simulink model "VTOL_v2_r2018b"  (R2018b)
settings: Solver=FixedStepAuto  StartTime=0.0  StopTime=inf  FixedStep=Ts  RelTol=1e-3  EnableMultiTasking=on
values from neighbouring files (symbols this model uses):
  deltaprops = 0*0.11/2    (= 0)    [VTOL_params.m]
  Ts = 1/10    (= 0.1)    [VTOL_params.m]
undefined symbols (not defined in the file or in its folder): dev, Main, pwm_output0
libraries: aerolibutil x7, px4uORBlib x4, pwm_sig_converters x4, px4Sensorslib x3, simulink x3, px4lib x1, sharedtransform x1
(part 1 of 2)
settings Model: SimulationMode=external  ExtModeTrigDuration=10  Creator=Robert  LastModifiedBy=Robert
settings SolverCC: PositivePriorityOrder=on
settings DataIOCC: SaveOutput=off  SignalLogging=off  DSMLogging=off  SaveTime=off
settings OptimizationCC: DefaultUnderspecifiedDataType=single  EnhancedBackFolding=on  PassReuseOutputArgsAs=Individual arguments  MaxStackSize=64  OptimizeBlockOrder=speed  DifferentSizesBufferReuse=on  OptimizationCustomize=off
settings DebuggingCC: ParameterTunabilityLossMsg=error
settings HardwareCC: ProdBitPerPointer=32  ProdBitPerSizeT=32  ProdBitPerPtrDiffT=32  ProdLargestAtomicInteger=Long  ProdLargestAtomicFloat=Double  ProdWordSize=32  ProdLongLongMode=on  ProdHWDeviceType=ARM Compatible->ARM Cortex
settings SFSimCC: MATLABDynamicMemAlloc=off
settings RTWCC: SystemTargetFile=ert.tlc  HardwareBoard=PX4 Pixhawk 1  TLCOptions="-aInlineSetEventsForThisBaseRateFcn=TLC_FALSE -aSuppressMultiTaskScheduler=TLC_FALSE  -aRateBasedStepFcn=0"  TemplateMakefile=ert_default_tmf  GenerateReport=on  Toolchain=GNU Tools for PX4 Autopilots  BuildConfiguration=Faster Runs  IncludeHyperlinkInReport=on  LaunchReport=on  TargetLang=C++  GenerateTraceInfo=on  GenerateTraceReport=on  GenerateTraceReportSl=on  GenerateTraceReportSf=on  GenerateTraceReportEml=on
settings CodeAppCC: ForceParamTrailComments=on  IgnoreCustomStorageClasses=off  OperatorAnnotations=on  SimulinkDataObjDesc=on  SFDataObjDesc=on  InsertBlockDesc=on

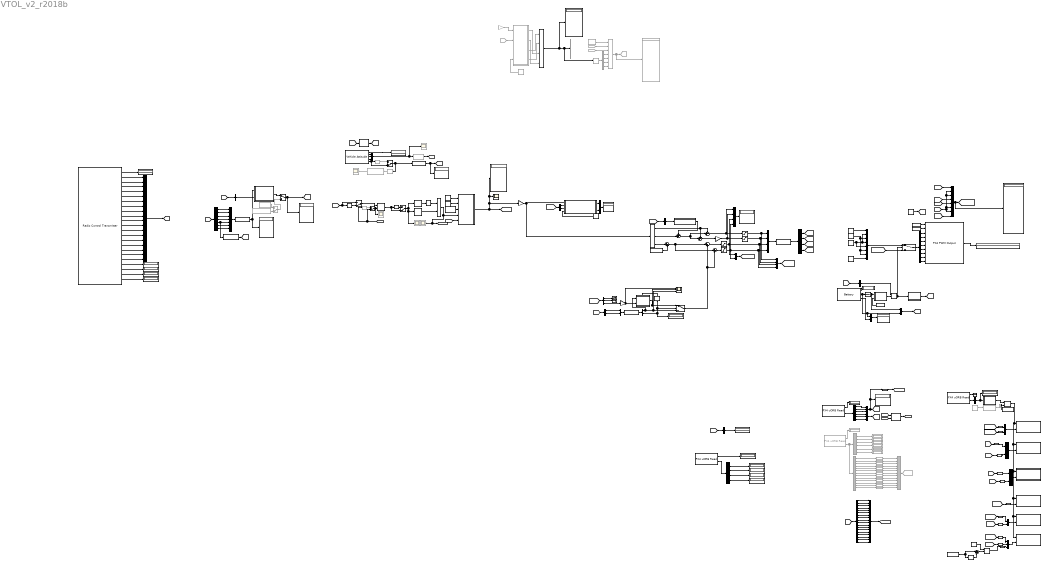
== system VTOL_v2_r2018b ==
  note: The PID parameters for roll/pitch on the single engine one
      | that works are approx
      | [0.6,0,0.015;
      |  0.6,0,0.015]
      |
      | That is, P/D = 40
  note: Some constant pitch torque offset
      | may be necessary due to c.g. z-offset. (No integrators in controller)
  note: Control Area
  note: Before Torque-Translator is used, lets make sure we can hover with this simple linear mixer.
      | Working around the hover point does not need the full range and thus complete non-linear controller.
      | Basic tuning is easier this way - less parameters to adjust.
  note: Part 2 of 2 of the heart of this project.
      | Once the Pixhawk is stable and hover works acceptable this part will be inserted, normalized to not
      | alter the behaviour too much at hover mode, and extend the responses to work well in flying and
      | transition mode as well.
  note: Old translator, only kept for code reference, will never be used.
  note: Crude, ad-hoc, altitude holder for the hover mode.
      | Far from perfect but does the job and frees up one hand to trim/adjust setting etc while hovering.
      | When not holding alt => Pass through
      | throttle stick to joint thrust.
  note: Generate reference quaternion from Transmitter inputs. Very crude reference now, but enough to test stability and do some small steps.
      | Verified in external mode with manual switches.
      |
      | The "mode" (bottom) selects absolute/rate mode
      | on input..
  note: Quaternion extraction from EKF.
      | Handedness verified with manual switches in external mode.
  note: Debug safety switch status
  note: lowpass filter batt voltage for
      | more accurate shutoffs
  note: 3V/cell in LiPo is absolutely the lowest allowed
  note: Make sure model runs at specified frequency
  note: Above (commented out) was a work-around before I got the
      | fixed code for the log block to log at every time step.
  note: Props may not be symmetrical, this offsets the thrust to compensate in that case.
  note: Emergency shutdown switch forces things into
      | off or neutral
  note: Inputs from RC
  note: Outputs, to Servos
  note: Emil Fresk paper on quaternion control, this is part 1 of 2 of the focus on this project. Originally a non-linear attitude controller for
      | multi-rotors, I am trying to use it as a controller for a VTOL fixed wing, non vectored along with a sensitivity normalizer
      | to allow a single controller for hover, transitioning and flying modes.
  note: If either manual emergency stop is pressed or voltage too low cut power.
  note: Logging to SD
  AND : Logic  IconShape=distinctive  AllPortsSameDT=off  OutDataTypeStr=boolean
  Battery : px4Sensorslib/Battery  voltage=on  current=off  remaining=on  warning=off  timestamp=off  sampleTime=Ts  BlockingMode=off  BlockTimeout=1e-3
      settings: SourceProductName=Embedded Coder Support Package for PX4 Autopilots
  Bus Creator : BusCreator  Inputs=18
  Bus Selector : BusSelector  OutputSignals=ch9_SC
  Bus Selector1 : BusSelector  OutputSignals=safety_switch_available,safety_off,override_available,override_enabled
  Bus Selector10 : BusSelector  Commented=on  OutputSignals=fix_type,satellites_used,lat,lon,alt,hdop,vdop,noise_per_ms,jamming_indicator,vel_m_s,vel_n_m_s,vel_e_m_s,vel_d_m_s
  Bus Selector11 : BusSelector  OutputSignals=ch10_SD
  Bus Selector12 : BusSelector  OutputSignals=ch5_S1
  Bus Selector13 : BusSelector  OutputSignals=safety_off
  Bus Selector2 : BusSelector  OutputSignals=ch5_S1
  Bus Selector3 : BusSelector  OutputSignals=ch1_thrust,ch2_Ail,ch3_Ele,ch4_Rud,ch8_SB,ch6_S2,ch7_SA
  Bus Selector6 : BusSelector  OutputSignals=x,y,z,vx,vy,vz
  Bus Selector7 : BusSelector  OutputSignals=ch1_thrust,ch2_Ail,ch3_Ele,ch4_Rud,ch5_S1,ch6_S2,ch7_SA,ch8_SB,ch9_SC,ch10_SD,ch11_SE,ch12_SF,ch13_SG,ch14_SH,ch15_LS,ch16_RS,ch17_MAX,ch18_MIN
  Bus Selector8 : BusSelector  Commented=on  OutputSignals=lat,lon,alt,satellites_used,hdop,vdop
  Bus Selector9 : BusSelector  OutputSignals=ch1_thrust,ch12_SF
  Cast To Boolean : DataTypeConversion  Commented=on  OutDataTypeStr=boolean
  Compare To Zero : simulink/Logic and Bit Operations/Compare To Zero  relop=>  OutDataTypeStr=boolean
  Constant : Constant  Value=logical(1)
  Constant1 : Constant  Value=logical(0)
  Constant10 : Constant  Value=1500  OutDataTypeStr=uint16
  Constant11 : Constant  Value=1500  OutDataTypeStr=uint16
  Constant12 : Constant  Value=1500  OutDataTypeStr=uint16  SampleTime=Ts
  Constant13 : Constant  Commented=on  Value=[cos(pi/4),0,sin(pi/4),0]  SampleTime=Ts
  Constant14 : Constant  Value=boolean(true)  SampleTime=Ts
  Constant16 : Constant  SampleTime=Ts
  Constant17 : Constant  Value=[2,4,1]'  VectorParams1D=off  SampleTime=Ts
  Constant2 : Constant  Commented=on  Value=[0,0,0]  OutDataTypeStr=single  SampleTime=Ts
  Constant3 : Constant  Commented=on  Value=0  SampleTime=Ts
  Constant4 : Constant  Value=0.015  SampleTime=Ts
  Constant5 : Constant  Value=0.6  SampleTime=Ts
  Constant6 : Constant  Value=[0,0,0]  SampleTime=Ts
  Constant7 : Constant  Value=1500  OutDataTypeStr=uint16
  Constant8 : Constant  Commented=on  Value=[1,0,0,0]  SampleTime=Ts
  Constant9 : Constant  Value=900  OutDataTypeStr=uint16
  CutoffVoltage : Constant  Value=3.0*3  OutDataTypeStr=single  SampleTime=Ts
  Data Type Conversion{4..16} (13 alike) : DataTypeConversion  Commented=on  OutDataTypeStr=single
  Data Type Conversion{2..3,17,20..26,28} (11 alike) : DataTypeConversion  OutDataTypeStr=single
  Data Type Conversion18 : DataTypeConversion  OutDataTypeStr=uint16
  Data Type Conversion19 : DataTypeConversion  OutDataTypeStr=uint16
  Data Type Conversion27 : DataTypeConversion  Commented=on  OutDataTypeStr=double
  Demux : Demux  Outputs=8
  Demux1 : Demux  Commented=on
  Demux4 : Demux  Commented=on
  Demux5 : Demux  Outputs=3
  Demux6 : Demux  Outputs=2
  Demux7 : Demux  Outputs=3
  Demux8 : Demux  Outputs=2
  Demux9 : Demux
  Digital Clock1 : DigitalClock  SampleTime=Ts
  Discrete Transfer Fcn : DiscreteTransferFcn  Numerator=[1-0.99]  Denominator=[1 -0.99]  SampleTime=Ts
  Display{,1..2,4..15,22,26..27,33..41} (27 alike) : Display
      Display9 settings: Format=binary (Stored Integer)
  Display{20..21,23,28..32} (8 alike) : Display  Commented=on
  Divide1 : Product  Inputs=*/
  From15 : From  Commented=on  GotoTag=w_bf
  From16 : From  Commented=on  GotoTag=q_bf
  From21 : From  Commented=on  GotoTag=states
  Gain1 : Gain  Commented=on  Gain=18
  Gain2 : Gain
  Gain3 : Gain  Gain=-1
  Gain4 : Gain  Gain=-1
  Goto11 : Goto  Commented=on  GotoTag=states
  Goto25 : Goto  Commented=on  GotoTag=GPSinfo
  MATLAB Function11 : MATLAB Function  TreatAsAtomicUnit=on
  MATLAB Function12 : MATLAB Function  TreatAsAtomicUnit=on
  MATLAB Function14 : MATLAB Function  TreatAsAtomicUnit=on
  MATLAB Function15 : MATLAB Function  TreatAsAtomicUnit=on
  MATLAB Function16 : MATLAB Function  TreatAsAtomicUnit=on
  MATLAB Function17 : MATLAB Function  TreatAsAtomicUnit=on
  MATLAB Function18 : MATLAB Function  TreatAsAtomicUnit=on
  Manual Switch{,1..3} (4 alike) : ManualSwitch  CurrentSetting=0
  Manual Switch4 : ManualSwitch
  Manual Switch5 : ManualSwitch  Commented=on  CurrentSetting=0
  Max : MinMax  Function=max  Inputs=2  OutDataTypeStr=uint16
  Memory : Memory  Commented=on  InheritSampleTime=on
  Memory2 : Memory  InheritSampleTime=on
  Multiply : Product
  Mux : Mux  Inputs=7
  Mux10 : Mux  Commented=on  Inputs=7
  Mux{11..12,17..20,22..23,26} (9 alike) : Mux  Inputs=2
  Mux13 : Mux  Commented=on  Inputs=13
  Mux14 : Mux  Inputs=8
  Mux{2,16,24,27} (4 alike) : Mux
  Mux21 : Mux  Inputs=8
  Mux{5..7,25} (4 alike) : Mux  Inputs=3
  Mux8 : Mux  Inputs=18
  PX4 PWM Output : px4lib/PX4 PWM Output  pwmDevice=Main (/dev/pwm_output0)  pwmChannel1_=on  pwmChannel2_=on  pwmChannel3_=on  pwmChannel4_=on  pwmChannel5_=on  pwmChannel6_=on  pwmChannel7_=on  pwmChannel8_=on  forceTerminateFailsafe=off  outputErrorStatus=on
      settings: SourceProductName=Embedded Coder Support Package for PX4 Autopilots
  PX4 SD Card Logger1 : Subsystem  mask(PX4 SD Card Logger){logfile=/fs/microsd/log, logfilename=qlogs, cacheflag=off, numRecs=250*60*60}
      mask prompts: logfile "Log Folder"; logfilename "Log File Name"; cacheflag "Cache in Memory"; numRecs "Maximum Record Count"
      mask help:
      | Log data to a specified file on the SD card
      |
      | The block accepts two inputs, enable and data. The incoming data is logged into the SD card when the enable signal is high and the number of data points logged is less than the Maximum Record Count specified.
      |
      | The specified folder should be present in the SD card for logging.
      |
      | If Cache in Memory is unchecked, the data is written to the SD card at every timestep.  If Cache in Memory is checked, data is cached in the memory and is written to SD card only when enable goes low or when the number of data points logged reaches the Maximum Record Count specified.
      mask init:
      | logname=uint8([logfile,'/',logfilename]);
      mask Help: eval('codertarget.internal.helpView(''px4'',''px4sdcardexample'')');
      mask Display:
      | fprintf([get_param(gcb,'logfile'),'/',get_param(gcb,'logfilename')])
      | port_label('input',1,'en')
      | port_label('input',2,'data')
  PX4 SD Card Logger2 : Subsystem  mask(PX4 SD Card Logger){logfile=/fs/microsd/log, logfilename=rc_and_servosignals, cacheflag=off, numRecs=250*60*60}
      mask prompts: logfile "Log Folder"; logfilename "Log File Name"; cacheflag "Cache in Memory"; numRecs "Maximum Record Count"
      mask help:
      | Log data to a specified file on the SD card
      |
      | The block accepts two inputs, enable and data. The incoming data is logged into the SD card when the enable signal is high and the number of data points logged is less than the Maximum Record Count specified.
      |
      | The specified folder should be present in the SD card for logging.
      |
      | If Cache in Memory is unchecked, the data is written to the SD card at every timestep.  If Cache in Memory is checked, data is cached in the memory and is written to SD card only when enable goes low or when the number of data points logged reaches the Maximum Record Count specified.
      mask init:
      | logname=uint8([logfile,'/',logfilename]);
      mask Help: eval('codertarget.internal.helpView(''px4'',''px4sdcardexample'')');
      mask Display:
      | fprintf([get_param(gcb,'logfile'),'/',get_param(gcb,'logfilename')])
      | port_label('input',1,'en')
      | port_label('input',2,'data')
  PX4 SD Card Logger3 : Subsystem  mask(PX4 SD Card Logger){logfile=/fs/microsd/log, logfilename=norm_sigs, cacheflag=off, numRecs=250*60*60}
      mask prompts: logfile "Log Folder"; logfilename "Log File Name"; cacheflag "Cache in Memory"; numRecs "Maximum Record Count"
      mask help:
      | Log data to a specified file on the SD card
      |
      | The block accepts two inputs, enable and data. The incoming data is logged into the SD card when the enable signal is high and the number of data points logged is less than the Maximum Record Count specified.
      |
      | The specified folder should be present in the SD card for logging.
      |
      | If Cache in Memory is unchecked, the data is written to the SD card at every timestep.  If Cache in Memory is checked, data is cached in the memory and is written to SD card only when enable goes low or when the number of data points logged reaches the Maximum Record Count specified.
      mask init:
      | logname=uint8([logfile,'/',logfilename]);
      mask Help: eval('codertarget.internal.helpView(''px4'',''px4sdcardexample'')');
      mask Display:
      | fprintf([get_param(gcb,'logfile'),'/',get_param(gcb,'logfilename')])
      | port_label('input',1,'en')
      | port_label('input',2,'data')
  PX4 SD Card Logger4 : Subsystem  mask(PX4 SD Card Logger){logfile=/fs/microsd/log, logfilename=MainLog, cacheflag=off, numRecs=250*60*60}
      mask prompts: logfile "Log Folder"; logfilename "Log File Name"; cacheflag "Cache in Memory"; numRecs "Maximum Record Count"
      mask help:
      | Log data to a specified file on the SD card
      |
      | The block accepts two inputs, enable and data. The incoming data is logged into the SD card when the enable signal is high and the number of data points logged is less than the Maximum Record Count specified.
      |
      | The specified folder should be present in the SD card for logging.
      |
      | If Cache in Memory is unchecked, the data is written to the SD card at every timestep.  If Cache in Memory is checked, data is cached in the memory and is written to SD card only when enable goes low or when the number of data points logged reaches the Maximum Record Count specified.
      mask init:
      | logname=uint8([logfile,'/',logfilename]);
      mask Help: eval('codertarget.internal.helpView(''px4'',''px4sdcardexample'')');
      mask Display:
      | fprintf([get_param(gcb,'logfile'),'/',get_param(gcb,'logfilename')])
      | port_label('input',1,'en')
      | port_label('input',2,'data')
  PX4 SD Card Logger5 : Subsystem  mask(PX4 SD Card Logger){logfile=/fs/microsd/log, logfilename=torques, cacheflag=off, numRecs=250*60*60}
      mask prompts: logfile "Log Folder"; logfilename "Log File Name"; cacheflag "Cache in Memory"; numRecs "Maximum Record Count"
      mask help:
      | Log data to a specified file on the SD card
      |
      | The block accepts two inputs, enable and data. The incoming data is logged into the SD card when the enable signal is high and the number of data points logged is less than the Maximum Record Count specified.
      |
      | The specified folder should be present in the SD card for logging.
      |
      | If Cache in Memory is unchecked, the data is written to the SD card at every timestep.  If Cache in Memory is checked, data is cached in the memory and is written to SD card only when enable goes low or when the number of data points logged reaches the Maximum Record Count specified.
      mask init:
      | logname=uint8([logfile,'/',logfilename]);
      mask Help: eval('codertarget.internal.helpView(''px4'',''px4sdcardexample'')');
      mask Display:
      | fprintf([get_param(gcb,'logfile'),'/',get_param(gcb,'logfilename')])
      | port_label('input',1,'en')
      | port_label('input',2,'data')
  PX4 SD Card Logger6 : Subsystem  mask(PX4 SD Card Logger){logfile=/fs/microsd/log, logfilename=volt_stop, cacheflag=off, numRecs=250*60*60}
      mask prompts: logfile "Log Folder"; logfilename "Log File Name"; cacheflag "Cache in Memory"; numRecs "Maximum Record Count"
      mask help:
      | Log data to a specified file on the SD card
      |
      | The block accepts two inputs, enable and data. The incoming data is logged into the SD card when the enable signal is high and the number of data points logged is less than the Maximum Record Count specified.
      |
      | The specified folder should be present in the SD card for logging.
      |
      | If Cache in Memory is unchecked, the data is written to the SD card at every timestep.  If Cache in Memory is checked, data is cached in the memory and is written to SD card only when enable goes low or when the number of data points logged reaches the Maximum Record Count specified.
      mask init:
      | logname=uint8([logfile,'/',logfilename]);
      mask Help: eval('codertarget.internal.helpView(''px4'',''px4sdcardexample'')');
      mask Display:
      | fprintf([get_param(gcb,'logfile'),'/',get_param(gcb,'logfilename')])
      | port_label('input',1,'en')
      | port_label('input',2,'data')
  PX4 uORB Read : px4uORBlib/PX4 uORB Read  uORBTopic=vehicle_local_position  sampleTime=Ts  BlockingMode=off  BlockTimeout=1e-3
      settings: SourceProductName=Embedded Coder Support Package for PX4 Autopilots
  PX4 uORB Read1 : px4uORBlib/PX4 uORB Read  uORBTopic=safety  sampleTime=Ts  BlockingMode=off  BlockTimeout=1e-3
      settings: SourceProductName=Embedded Coder Support Package for PX4 Autopilots
  PX4 uORB Read2 : px4uORBlib/PX4 uORB Read  Commented=on  uORBTopic=vehicle_gps_position  sampleTime=0.004  BlockingMode=off  BlockTimeout=1e-3
      settings: SourceProductName=Embedded Coder Support Package for PX4 Autopilots
  PX4 uORB Read3 : px4uORBlib/PX4 uORB Read  uORBTopic=safety  sampleTime=Ts  BlockingMode=off  BlockTimeout=1e-3
      settings: SourceProductName=Embedded Coder Support Package for PX4 Autopilots
  PropOffset : Constant  Value=deltaprops  OutDataTypeStr=single  SampleTime=Ts
  Pulse Generator : DiscretePulseGenerator  Commented=on  SampleTime=Ts
  Quaternion Conjugate1 : aerolibutil/Quaternion Conjugate
      settings: SourceProductName=Aerospace Blockset  SourceProductBaseCode=AE
  Quaternion Conjugate10 : aerolibutil/Quaternion Conjugate
      settings: SourceProductName=Aerospace Blockset  SourceProductBaseCode=AE
  Quaternion Conjugate2 : aerolibutil/Quaternion Conjugate  Commented=on
      settings: SourceProductName=Aerospace Blockset  SourceProductBaseCode=AE
  Quaternion Conjugate7 : aerolibutil/Quaternion Conjugate  Commented=on
      settings: SourceProductName=Aerospace Blockset  SourceProductBaseCode=AE
  Quaternion Conjugate8 : aerolibutil/Quaternion Conjugate
      settings: SourceProductName=Aerospace Blockset  SourceProductBaseCode=AE
  Quaternion Multiplication : aerolibutil/Quaternion Multiplication
  Quaternion Rotation4 : aerolibutil/Quaternion Rotation
  Quaternions to Rotation Angles1 : sharedtransform/Quaternions to Rotation Angles  Commented=on  rotationOrder=ZYX  aMode=aMode
      settings: SourceProductBaseCode=AE
  Radio Control Transmitter : px4Sensorslib/Radio Control Transmitter  channel1=on  channel2=on  channel3=on  channel4=on  channel5=on  channel6=on  channel7=on  channel8=on  channel9=on  channel10=on  channel11=on  channel12=on  channel13=on  channel14=on  channel15=on  channel16=on  channel17=on  channel18=on  channel_count=on  rssi=on  rc_input_source=on  timestamp_last_signal=on  time_stamp=off  sampleTime=Ts  BlockingMode=off  BlockTimeout=5
      settings: SourceProductName=Embedded Coder Support Package for PX4 Autopilots
  Saturation{,1..3} (4 alike) : Saturate  UpperLimit=1  LowerLimit=-1
  Scope : Scope  NumInputPorts=3
  Scope{4..6,25,35} (5 alike) : Scope  Commented=on
  Scope7 : Scope
  Selector2 : Selector  IndexMode=Zero-based  InputPortWidth=4  IndexOptions=Index vector (dialog)  Indices=[0 ]  OutputSizes=1
  Selector3 : Selector  IndexMode=Zero-based  InputPortWidth=4  IndexOptions=Index vector (dialog)  Indices=[1:3]  OutputSizes=1
  Sign : Signum
  Signal Specification1 : SignalSpecification  OutDataTypeStr=single
  Subsystem : Subsystem
  Sum2 : Sum  Inputs=-+|
  Sum3 : Sum  Inputs=++|
  Sum4 : Sum  Inputs=|++
  Sum5 : Sum  Inputs=|-+
  Sum6 : Sum  Inputs=++|
  Sum7 : Sum  Inputs=|++
  Sum9 : Sum  Inputs=|+-
  Switch : Switch  Criteria=u2 > Threshold
  Switch1 : Switch  Criteria=u2 > Threshold  Threshold=1300
  Terminator : Terminator
  Terminator1 : Terminator
  Terminator2 : Terminator
  TorqueTranslator : MATLAB Function  Commented=on  TreatAsAtomicUnit=on
  Transfer Fcn First Order1 : simulink/Discrete/Transfer Fcn First Order  Commented=through  PoleZ=0.9  ICPrevOutput=0.0  DoSatur=off
      settings: SourceProductName=Simulink
  Vehicle Attitude1 : px4Sensorslib/Vehicle Attitude  rollRate=on  pitchRate=on  yawRate=on  quaternion=on  uorbTimeStamp=off  BlockingMode=off  BlockTimeout=0.001  sampleTime=Ts
      settings: SourceProductName=Embedded Coder Support Package for PX4 Autopilots
  pwm2sig : pwm_sig_converters/pwm2sig  SystemSampleTime=-1
  pwm2sig1 : pwm_sig_converters/pwm2sig  SystemSampleTime=-1
  pwm2sig2 : pwm_sig_converters/pwm2sig  SystemSampleTime=-1
  sig2pwm : pwm_sig_converters/sig2pwm  SystemSampleTime=-1
  wires:
  Demux1/4 -> Mux10/7
  Quaternion Conjugate7/1 -> Manual Switch/1
  Demux6/2 -> Display37/1, Switch/2, Compare To Zero/1
  Bus Selector7/10 -> Mux8/10  "<ch10_SD>"
  Sum3/1 -> Gain3/1
  Demux7/2 -> Terminator1/1
  Multiply/1 -> [axis_err], Scope4/1, MATLAB Function11/4(angErr)
  Battery/3 -> Mux22/2
  Demux5/1 -> Sum2/1, Sum3/1  "tao_x"
  [rc_bus] -> Bus Selector11/1
  Switch1/1 -> Demux/1
  Compare To Zero/1 -> Subsystem/Enable
  Battery/2 -> Discrete Transfer Fcn/1, Mux26/2, Mux22/1
  Demux/8 -> PX4 PWM Output/10
  Data Type Conversion8/1 -> Mux13/5
  Constant11/1 -> Mux21/8
  Mux2/1 -> Memory/1, Demux4/1, Display10/1
  Bus Selector/1 -> Display/1  "<ch9_SC>"
  Demux9/2 -> [ElevonR]
  Radio Control Transmitter/16 -> Bus Creator/15  "ch15_LS"
  Demux1/2 -> Mux10/5
  Constant7/1 -> Mux21/1
  Demux/1 -> PX4 PWM Output/3
  Constant9/1 -> Mux21/2, Mux21/4, Mux21/5
  Bus Selector7/2 -> Mux8/2  "<ch2_Ail>"
  Radio Control Transmitter/8 -> Bus Creator/7  "ch7_SA"
  Quaternion Multiplication/1 -> Quaternion Conjugate10/1, Manual Switch3/2  "qerr_wf"
  Demux7/3 -> Gain4/1
  Demux9/4 -> [ThrustR]
  Constant6/1 -> MATLAB Function14/4(v)
  [ServoSignals] -> Switch1/3
  Bus Selector10/2 -> Data Type Conversion5/1  "<satellites_used>"
  Mux20/1 -> Display38/1
  Max/1 -> MATLAB Function18/1(u), Switch1/2
  Sum6/1 -> Sum3/2, Sum2/2
  Bus Selector7/3 -> Mux8/3  "<ch3_Ele>"
  Bus Selector10/6 -> Data Type Conversion9/1  "<hdop>"
  Data Type Conversion6/1 -> Mux13/3
  Subsystem/1("throttle ") -> Switch/1, Scope/2
  Constant10/1 -> Mux21/7, Mux21/6, Mux21/3
  Bus Selector6/5 -> Mux7/2  "<vy>"
  MATLAB Function15/1(stopsig) -> Max/2
  Demux8/1 -> MATLAB Function14/2(u_omegaL)
  Bus Selector3/5 -> pwm2sig2/1, Mux/5  "<ch8_SB>"
  Radio Control Transmitter/19 -> Bus Creator/18  "ch18_MIN"
  Data Type Conversion9/1 -> Mux13/6
  Bus Selector8/4 -> Display21/1  "<satellites_used>"
  TorqueTranslator/3(u_deltaL) -> Mux2/1  "uWL"
  Bus Selector10/10 -> Data Type Conversion13/1  "<vel_m_s>"
  Manual Switch1/1 -> Quaternion Multiplication/1
  Bus Selector6/1 -> Mux5/1  "<x>"
  PX4 PWM Output/1 -> Display9/1
  Gain3/1 -> Mux16/2, Saturation1/1
  Gain2/1 -> MATLAB Function14/1(tao), Demux5/1
  Bus Selector3/6 -> Mux/6  "<ch6_S2>"
  Bus Selector9/1 -> Mux18/1  "<ch1_thrust>"
  Switch/1 -> Sum4/2, Sum5/2
  Mux22/1 -> Display39/1
  Bus Selector11/1 -> Max/1  "<ch10_SD>"
  Radio Control Transmitter/21 -> Display12/1
  Demux6/1 -> Subsystem/1(throttle), Switch/3, Scope/3
  Bus Selector1/3 -> Display6/1  "<override_available>"
  Demux/4 -> PX4 PWM Output/6
  Demux8/2 -> MATLAB Function14/3(u_omegaR)
  Data Type Conversion7/1 -> Mux13/4
  [u_omegas] -> Demux8/1
  Bus Selector10/9 -> Data Type Conversion12/1  "<jamming_indicator>"
  [q_wf] -> Manual Switch/2, Quaternion Conjugate7/1  "qerr_bf"
  Sum7/1 -> Sum5/1, Sum4/1
  Demux/3 -> PX4 PWM Output/5
  Manual Switch4/1 -> [q_ref], Display36/1
  [Position] -> Demux7/1
  Constant2/1 -> Mux10/1
  Bus Selector8/1 -> Display29/1  "<lat>"
  Mux21/1 -> Switch1/1
  Manual Switch3/1 -> Scope35/1, Selector3/1, Selector2/1
  Mux19/1 -> [u_omegas]
  [w_bf] -> MATLAB Function11/5(w)
  Bus Selector7/8 -> Mux8/8  "<ch8_SB>"
  Sign/1 -> Multiply/1  "rotdir"
  Data Type Conversion16/1 -> Mux13/13
  Gain4/1 -> Scope/1, Subsystem/2(alt)
  Vehicle Attitude1/5 -> Manual Switch2/2, Quaternion Conjugate2/1
  Vehicle Attitude1/4 -> Mux6/3
  Radio Control Transmitter/6 -> Bus Creator/5  "ch5_S1"
  [ElevonR] -> Mux14/1
  TorqueTranslator/4(u_deltaR) -> Mux2/2  "udeltaL"
  Vehicle Attitude1/2 -> Mux6/1
  Bus Selector1/1 -> Display4/1  "<safety_switch_available>"
  Quaternion Conjugate1/1 -> [q_bf]
  Constant17/1 -> MATLAB Function11/3(axisgains)
  PX4 uORB Read1/2 -> Bus Selector1/1
  pwm2sig1/1 -> MATLAB Function12/1(sticks), Display35/1
  [rc_bus] -> Bus Selector3/1
  Demux9/3 -> [ThrustL]
  Bus Selector10/11 -> Data Type Conversion14/1  "<vel_n_m_s>"
  Bus Selector6/4 -> Mux7/1  "<vx>"
  Bus Selector3/3 -> Mux/3  "<ch3_Ele>"
  Bus Selector3/1 -> Mux/1  "<ch1_thrust>"
  Bus Selector10/8 -> Data Type Conversion11/1  "<noise_per_ms>"
  Demux9/1 -> [ElevonL]
  Data Type Conversion14/1 -> Mux13/11
  Bus Selector10/12 -> Data Type Conversion15/1  "<vel_e_m_s>"
  Bus Selector7/15 -> Mux8/15  "<ch15_LS>"
  Data Type Conversion12/1 -> Mux13/9
  Data Type Conversion13/1 -> Mux13/10
  Bus Selector7/9 -> Mux8/9  "<ch9_SC>"
  [ThrustL] -> Mux14/5
  Data Type Conversion10/1 -> Mux13/7
  Data Type Conversion5/1 -> Mux13/2
  Demux/6 -> PX4 PWM Output/8
  Selector3/1 -> Multiply/2  "axiserr"
  Demux/7 -> PX4 PWM Output/9
  Mux7/1 -> [v_wf]
  Mux14/1 -> Display8/1, [ServoSignals]
  [Others] -> Mux14/2, Mux14/3, Mux14/6, Mux14/7
  Bus Selector7/12 -> Mux8/12  "<ch12_SF>"
  Radio Control Transmitter/3 -> Bus Creator/2  "ch2_Ail"
  Bus Selector7/14 -> Mux8/14  "<ch14_SH>"
  Bus Selector7/11 -> Mux8/11  "<ch11_SE>"
  Radio Control Transmitter/23 -> Display13/1
  Bus Selector10/1 -> Data Type Conversion4/1  "<fix_type>"
  [rc_bus] -> Bus Selector7/1
  Bus Selector7/6 -> Mux8/6  "<ch6_S2>"
  Bus Selector10/13 -> Data Type Conversion16/1  "<vel_d_m_s>"
  TorqueTranslator/2(u_omegaR) -> Mux2/4
  Bus Selector7/7 -> Mux8/7  "<ch7_SA>"
  [q_wf] -> Quaternion Conjugate1/1
  Manual Switch/1 -> Scope25/1, Quaternion Multiplication/2
  Bus Selector7/18 -> Mux8/18  "<ch18_MIN>"
  Mux16/1 -> Display33/1
  Selector2/1 -> Sign/1  "q0"
  Sum2/1 -> Mux16/1, Saturation/1
  From16/1 -> Mux10/3  "q"
  [q_ref] -> Manual Switch1/1, Quaternion Conjugate8/1
  Vehicle Attitude1/3 -> Mux6/2
  Constant4/1 -> MATLAB Function11/2(D)
  Gain1/1 -> TorqueTranslator/1(u_jointT)
  Data Type Conversion17/1 -> [Position]
  Constant5/1 -> MATLAB Function11/1(P)
  MATLAB Function11/1(taos) -> Display27/1, Scope7/1, Gain2/1, [torques]
  PX4 uORB Read1/1 -> Display1/1
  [v_wf] -> Quaternion Rotation4/2
  Bus Selector7/4 -> Mux8/4  "<ch4_Rud>"
  Bus Selector7/17 -> Mux8/17  "<ch17_MAX>"
  Bus Selector1/2 -> Display5/1  "<safety_off>"
  Sum5/1 -> Saturation3/1
  Bus Selector9/2 -> Mux18/2  "<ch12_SF>"
  Radio Control Transmitter/17 -> Bus Creator/16  "ch16_RS"
  Constant3/1 -> TorqueTranslator/4(pitchoffset)
  From21/1 -> TorqueTranslator/2(states)
  Demux/2 -> PX4 PWM Output/4
  Bus Selector7/16 -> Mux8/16  "<ch16_RS>"
  Memory/1 -> Demux1/1
  Data Type Conversion11/1 -> Mux13/8
  Radio Control Transmitter/11 -> Bus Creator/10  "ch10_SD"
  Sum4/1 -> Saturation2/1
  From15/1 -> Mux10/2  "w"
  TorqueTranslator/1(u_omegaL) -> Mux2/3  "uWL"
  Radio Control Transmitter/20 -> Display11/1
  [ElevonL] -> Mux14/8
  MATLAB Function14/2(u_deltaR) -> Mux20/2
  pwm2sig2/1 -> [mode]
  PX4 uORB Read/1 -> Display34/1
  [ThrustR] -> Mux14/4
  Bus Selector10/4 -> Data Type Conversion7/1  "<lon>"
  Bus Selector3/2 -> Mux/2  "<ch2_Ail>"
  Data Type Conversion4/1 -> Mux13/1
  Quaternion Rotation4/1 -> [v_bf]
  Radio Control Transmitter/14 -> Bus Creator/13  "ch13_SG"
  Signal Specification1/1 -> Display22/1, [q_wf]
  Vehicle Attitude1/1 -> Display26/1
  Bus Selector6/3 -> Mux5/3  "<z>"
  Bus Selector8/2 -> Display30/1  "<lon>"
  PX4 uORB Read/2 -> Bus Selector6/1
  CutoffVoltage/1 -> MATLAB Function15/2(cutoff)
  Radio Control Transmitter/22 -> Display15/1
  Radio Control Transmitter/10 -> Bus Creator/9  "ch9_SC"
  Radio Control Transmitter/15 -> Bus Creator/14  "ch14_SH"
  Radio Control Transmitter/13 -> Bus Creator/12  "ch12_SF"
  Bus Selector7/1 -> Mux8/1  "<ch1_thrust>"
  Radio Control Transmitter/18 -> Bus Creator/17  "ch17_MAX"
  Battery/1 -> Display40/1
  [q_bf] -> Quaternion Rotation4/1
  Mux8/1 -> [RC_inputs]
  Bus Selector10/3 -> Data Type Conversion6/1  "<lat>"
  PX4 uORB Read2/1 -> Display32/1
  Mux18/1 -> pwm2sig/1
  MATLAB Function14/1(u_deltaL) -> Mux20/1
  Radio Control Transmitter/4 -> Bus Creator/3  "ch3_Ele"
  Demux7/1 -> Terminator/1
  Constant1/1 -> PX4 PWM Output/2
  Bus Creator/1 -> [rc_bus]
  Bus Selector1/4 -> Display7/1  "<override_enabled>"
  Bus Selector6/6 -> Mux7/3  "<vz>"
  Radio Control Transmitter/5 -> Bus Creator/4  "ch4_Rud"
  Constant/1 -> PX4 PWM Output/1
  Constant12/1 -> [Others]
  Bus Selector7/5 -> Mux8/5  "<ch5_S1>"
  Demux1/1 -> Mux10/4
  Radio Control Transmitter/1 -> Display14/1
  Radio Control Transmitter/9 -> Bus Creator/8  "ch8_SB"
  [rc_bus] -> Bus Selector/1
  PX4 uORB Read2/2 -> Bus Selector10/1, Bus Selector8/1
  Mux/1 -> pwm2sig1/1
  Radio Control Transmitter/2 -> Bus Creator/1  "ch1_thrust"
  Quaternion Conjugate8/1 -> Manual Switch1/2
  Bus Selector10/5 -> Data Type Conversion8/1  "<alt>"
  Demux1/3 -> Mux10/6
  Bus Selector6/2 -> Mux5/2  "<y>"
  Mux13/1 -> Goto25/1
  Radio Control Transmitter/12 -> Bus Creator/11  "ch11_SE"
  Bus Selector7/13 -> Mux8/13  "<ch13_SG>"
  Mux5/1 -> Data Type Conversion17/1, Display2/1, [r_wf]
  pwm2sig/1 -> Demux6/1
  Mux10/1 -> Display31/1, Goto11/1
  Radio Control Transmitter/7 -> Bus Creator/6  "ch6_S2"
  Bus Selector10/7 -> Data Type Conversion10/1  "<vdop>"
  Data Type Conversion15/1 -> Mux13/12
  [rc_bus] -> Bus Selector9/1
  Bus Selector3/4 -> Mux/4  "<ch4_Rud>"
  Bus Selector8/5 -> Display23/1  "<hdop>"
  Demux/5 -> PX4 PWM Output/7
  Bus Selector8/3 -> Display28/1  "<alt>"
  Bus Selector8/6 -> Display20/1  "<vdop>"
  Saturation/1 -> Mux27/1, Mux24/1
  Saturation1/1 -> Mux27/2, Mux24/2
  Saturation2/1 -> Mux19/1, Mux16/3, Mux27/3, Mux24/3
  Saturation3/1 -> Mux19/2, Mux16/4, Mux27/4, Mux24/4
  Demux5/2 -> Sum6/2  "tao_y"
  MATLAB Function16/1(offset) -> Sum6/1
  Bus Selector3/7 -> Mux/7  "<ch7_SA>"
  [rc_bus] -> Bus Selector2/1
  Bus Selector2/1 -> MATLAB Function12/2(offset_stick)  "<ch5_S1>"
  Transfer Fcn First Order1/1 -> [w_bf]
  Bus Selector12/1 -> MATLAB Function16/1(offset_stick)  "<ch5_S1>"
  [rc_bus] -> Bus Selector12/1
  PX4 uORB Read3/2 -> Bus Selector13/1
  Bus Selector13/1 -> MATLAB Function17/1(u), Display41/1  "<safety_off>"
  Mux24/1 -> [norm_sigs]
  Demux5/3 -> Sum7/1  "tao_z"
  PropOffset/1 -> Sum7/2
  MATLAB Function17/1(y) -> AND/1
  [q_ref] -> Data Type Conversion21/1
  Data Type Conversion23/1 -> Mux23/1
  [torques] -> Data Type Conversion23/1
  [mode] -> Data Type Conversion2/1
  [RC_inputs] -> Data Type Conversion18/1
  Data Type Conversion2/1 -> Mux12/1
  [ServoSignals] -> Data Type Conversion19/1
  Data Type Conversion18/1 -> Mux11/1
  [axis_err] -> Data Type Conversion25/1
  [q_wf] -> Data Type Conversion3/1
  Data Type Conversion19/1 -> Mux11/2
  [Position] -> Data Type Conversion20/1
  [norm_sigs] -> Data Type Conversion24/1
  Data Type Conversion20/1 -> Mux12/2
  Mux17/1 -> PX4 SD Card Logger1/2(Data)
  Mux11/1 -> PX4 SD Card Logger2/2(Data)
  Mux23/1 -> PX4 SD Card Logger5/2(Data)
  Data Type Conversion24/1 -> PX4 SD Card Logger3/2(Data)
  Data Type Conversion21/1 -> Mux17/2
  Mux12/1 -> PX4 SD Card Logger4/2(Data)
  Data Type Conversion3/1 -> Mux17/1
  Data Type Conversion25/1 -> Mux23/2
  Pulse Generator/1 -> Cast To Boolean/1
  Cast To Boolean/1 -> ?
  Mux25/1 -> PX4 SD Card Logger6/2(Data)
  Data Type Conversion26/1 -> Mux25/2
  AND/1 -> PX4 SD Card Logger6/1(En), PX4 SD Card Logger5/1(En), PX4 SD Card Logger3/1(En), PX4 SD Card Logger1/1(En), PX4 SD Card Logger4/1(En), PX4 SD Card Logger2/1(En)
  [stop] -> Data Type Conversion26/1
  Data Type Conversion22/1 -> Mux25/1
  [volt] -> Data Type Conversion22/1
  MATLAB Function18/1(y) -> [stop]
  PX4 uORB Read3/1 -> Terminator2/1
  Discrete Transfer Fcn/1 -> MATLAB Function15/1(voltage), Mux26/1
  Mux26/1 -> [volt]
  Quaternion Conjugate2/1 -> Manual Switch2/1
  Manual Switch2/1 -> Data Type Conversion27/1, Signal Specification1/1
  Mux6/1 -> Scope5/1, Transfer Fcn First Order1/1
  Quaternions to Rotation Angles1/1 -> Scope6/1
  Data Type Conversion27/1 -> Quaternions to Rotation Angles1/1
  Quaternion Conjugate10/1 -> Manual Switch3/1
  Manual Switch5/1 -> Manual Switch4/2
  MATLAB Function12/1(q_ref) -> Manual Switch4/1
  Constant13/1 -> Manual Switch5/2
  Constant8/1 -> Manual Switch5/1
  Constant14/1 -> AND/2
  Divide1/1 -> Data Type Conversion28/1
  Sum9/1 -> Divide1/2
  Constant16/1 -> Divide1/1
  Memory2/1 -> Sum9/2
  Digital Clock1/1 -> Sum9/1, Memory2/1
  Data Type Conversion28/1 -> Mux25/3
  sig2pwm/1 -> Demux9/1
  Mux27/1 -> sig2pwm/1

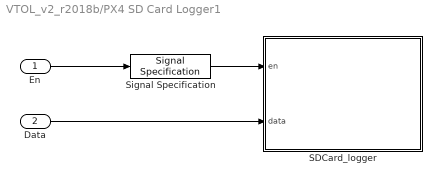
== system VTOL_v2_r2018b/PX4 SD Card Logger1 ==
  En : Inport
  Data : Inport  Port=2
  SDCard_logger : MATLAB Function  TreatAsAtomicUnit=on
  Signal Specification : SignalSpecification  OutDataTypeStr=boolean
  wires:
  Signal Specification/1 -> SDCard_logger/1(en)
  En/1 -> Signal Specification/1
  Data/1 -> SDCard_logger/2(data)

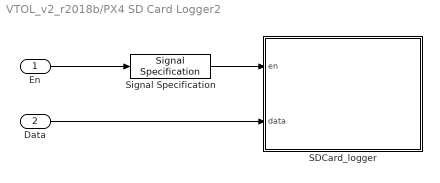
== system VTOL_v2_r2018b/PX4 SD Card Logger2 ==
  En : Inport
  Data : Inport  Port=2
  SDCard_logger : MATLAB Function  TreatAsAtomicUnit=on
  Signal Specification : SignalSpecification  OutDataTypeStr=boolean
  wires:
  Signal Specification/1 -> SDCard_logger/1(en)
  En/1 -> Signal Specification/1
  Data/1 -> SDCard_logger/2(data)

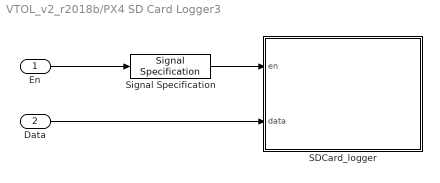
== system VTOL_v2_r2018b/PX4 SD Card Logger3 ==
  En : Inport
  Data : Inport  Port=2
  SDCard_logger : MATLAB Function  TreatAsAtomicUnit=on
  Signal Specification : SignalSpecification  OutDataTypeStr=boolean
  wires:
  Signal Specification/1 -> SDCard_logger/1(en)
  En/1 -> Signal Specification/1
  Data/1 -> SDCard_logger/2(data)

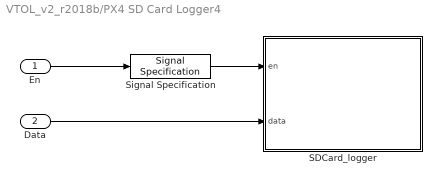
== system VTOL_v2_r2018b/PX4 SD Card Logger4 ==
  En : Inport
  Data : Inport  Port=2
  SDCard_logger : MATLAB Function  TreatAsAtomicUnit=on
  Signal Specification : SignalSpecification  OutDataTypeStr=boolean
  wires:
  Signal Specification/1 -> SDCard_logger/1(en)
  En/1 -> Signal Specification/1
  Data/1 -> SDCard_logger/2(data)

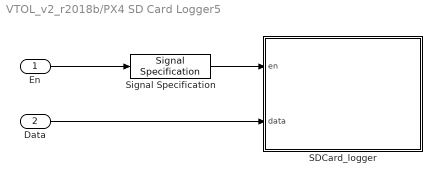
== system VTOL_v2_r2018b/PX4 SD Card Logger5 ==
  En : Inport
  Data : Inport  Port=2
  SDCard_logger : MATLAB Function  TreatAsAtomicUnit=on
  Signal Specification : SignalSpecification  OutDataTypeStr=boolean
  wires:
  Signal Specification/1 -> SDCard_logger/1(en)
  En/1 -> Signal Specification/1
  Data/1 -> SDCard_logger/2(data)

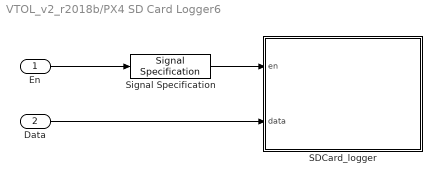
== system VTOL_v2_r2018b/PX4 SD Card Logger6 ==
  En : Inport
  Data : Inport  Port=2
  SDCard_logger : MATLAB Function  TreatAsAtomicUnit=on
  Signal Specification : SignalSpecification  OutDataTypeStr=boolean
  wires:
  Signal Specification/1 -> SDCard_logger/1(en)
  En/1 -> Signal Specification/1
  Data/1 -> SDCard_logger/2(data)

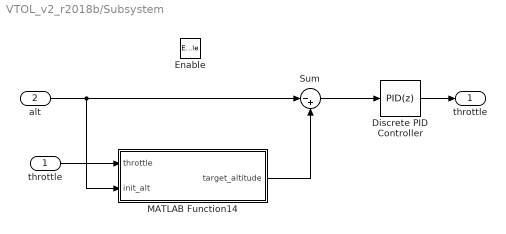
== system VTOL_v2_r2018b/Subsystem ==
  throttle : Inport
  alt : Inport  Port=2
  Enable : EnablePort  StatesWhenEnabling=reset
  Discrete PID Controller : simulink/Continuous/PID Controller  Controller=PID  Form=Parallel  TimeDomain=Discrete-time  SampleTime=-1  IntegratorMethod=Forward Euler  FilterMethod=Forward Euler  ControllerParametersSource=internal  P=0.5  I=0.01  D=0.1  UseFilter=off  N=100  TunerSelectOption=Transfer Function Based (PID Tuner App)  InitialConditionSource=internal  InitialConditionForIntegrator=0  InitialConditionForFilter=0  DifferentiatorICPrevScaledInput=0  ExternalReset=none  TrackingMode=off  Kt=1  LimitOutput=on  UpperSaturationLimit=1  LowerSaturationLimit=-1  LinearizeAsGain=off  AntiWindupMode=none  Kb=1  POutMin=[]  POutMax=[]  IOutMin=[]  IOutMax=[]  DOutMin=[]  DOutMax=[]  NOutMin=[]  NOutMax=[]  SumOutMin=[]  SumOutMax=[]  SaturationOutMin=[]  SaturationOutMax=[]  PParamMin=[]  PParamMax=[]  IParamMin=[]  IParamMax=[]  DParamMin=[]  DParamMax=[]  NParamMin=[]  NParamMax=[]  KbParamMin=[]  KbParamMax=[]  KtParamMin=[]  KtParamMax=[]  KbOutMin=[]  KbOutMax=[]  KtOutMin=[]  KtOutMax=[]  IntegratorOutMin=[]  IntegratorOutMax=[]  FilterOutMin=[]  FilterOutMax=[]  SumI1OutMin=[]  SumI1OutMax=[]  SumI2OutMin=[]  SumI2OutMax=[]  SumI3OutMin=[]  SumI3OutMax=[]  SumI4OutMin=[]  SumI4OutMax=[]  SumDOutMin=[]  SumDOutMax=[]  DifferentiatorOutMin=[]  DifferentiatorOutMax=[]  FilterDiffOutCoefMin=[]  FilterDiffOutCoefMax=[]  ReciprocalOutMin=[]  ReciprocalOutMax=[]  SumDenOutMin=[]  SumDenOutMax=[]  SumNumOutMin=[]  SumNumOutMax=[]  DivideOutMin=[]  DivideOutMax=[]  IntegratorContinuousStateAttributes=''  IntegratorStateMustResolveToSignalObject=off  IntegratorRTWStateStorageClass=Auto  FilterContinuousStateAttributes=''  FilterStateMustResolveToSignalObject=off  FilterRTWStateStorageClass=Auto  ParallelPVariant=InternalParameters  IdealPVariant=Disabled  IVariant=InternalParameters  DVariant=InternalParameters  IntegratorVariant=Discrete  SatVariant=Enabled  AWVariant=Passthrough  PCopyVariant=Disabled  TRVariant=Disabled  FdbkBlocksVariant=Forward  IdealPFdbkVariant=Disabled  SatFdbkVariant=Disabled  DerivativeFilterVariant=Differentiator  NVariant=Passthrough  NCopyVariant=Disabled_SignalSpec  FilterICVariant=InternalICsDifferentiator  IntegratorICVariant=InternalICs  ExternalResetVariant=Disabled  TRSumVariant=Passthrough  SumFdbkVariant=Disabled  SumVariant=Sum_PID
  MATLAB Function14 : MATLAB Function  TreatAsAtomicUnit=on
  Sum : Sum  Inputs=|-+
  "throttle " : Outport
  wires:
  throttle/1 -> MATLAB Function14/1(throttle)
  MATLAB Function14/1(target_altitude) -> Sum/2
  Sum/1 -> Discrete PID Controller/1
  Discrete PID Controller/1 -> "throttle "/1
  alt/1 -> MATLAB Function14/2(init_alt), Sum/1

== matlab function VTOL_v2_r2018b/PX4 SD Card Logger2/SDCard_logger ==
  data: en input boolean; data input; logname parameter uint8; cacheflag parameter boolean; numRecs parameter uint32
%% PX4 SD Card Logger
% Note: All data needs to be of the same type (e.g. double)
% Header information format:
%           String "MWLOG"
%           Time/Date 4 bytes (time())
%           Number of Signals per record Logged 1 byte (256 max)
%           Data Type of Signals Logged  1 byte (1-10)
%           Number of bytes per record 2 bytes (65535 max)
% This does NOT include the number of data sets logged.
% i.e. The Reader is responsible for reading until EOF.
% Steve Kuznicki
% Copyright 2018 The MathWorks, Inc.

function SDCard_logger(en, data, logname, cacheflag, numRecs)

persistent fp count elem_size vect_size datastore timestore count_prev

if coder.target('Rtw')
    
    coder.cinclude('<stdio.h>');
    coder.cinclude('<time.h>');
    
    if coder.target('Rtw')
        coder.cinclude('<drivers/drv_hrt.h>');
    end
    
    if coder.target('Rtw')
        timestamp=coder.opaque('uint64_t');
        timestamp=coder.ceval('hrt_absolute_time');
    else
        timestamp = uint64(0);
    end
    
    if isempty(count)
        count = uint32(0);
        count_prev=count;
        fp = coder.opaque('FILE*', 'NULL');
        if cacheflag == true
            datastore = zeros(numRecs*uint32(coder.const(numel(data))), 1, 'like', data);
            timestore=uint64(zeros(numRecs, 1));
        end
        
        [elsize, eltype] = get_elem_size(data);
        elem_size = coder.const(uint16(elsize));
        elem_type = coder.const(uint8(eltype));
        vect_size = coder.const(uint8(numel(data)));
        coder.ceval('printf',['OPENING file %s vect_size %d elem_size %d numRecs %d %c' uint8(0)], ...
            [logname,'.bin', int8(0)], uint32(vect_size), uint32(elem_size), uint32(numRecs), uint8(10));
        fp = coder.ceval('fopen', [logname,'.bin', int8(0)], ['wb', int8(0)]);
        
        % Write header information here
        % header token + version
        mlStrVer = 'MWLOG';
        coder.ceval('fwrite', coder.rref(mlStrVer), uint32(1), length(mlStrVer), fp);
        % date/time
        tm = uint32(0);
        tmptr = uint32(0);
        tm = coder.ceval('time',coder.wref(tmptr));
        coder.ceval('fwrite', coder.rref(tm), uint32(4), uint32(1), fp);
        % number of elements in each record
        coder.ceval('fwrite', coder.rref(vect_size), uint32(1), uint32(1), fp);
        % data type of the elements
        coder.ceval('fwrite', coder.rref(elem_type), uint32(1), uint32(1), fp);
        % size of each record in bytes
        recSize = elem_size * uint16(vect_size);
        coder.ceval('fwrite', coder.rref(recSize), uint32(2), uint32(1), fp);
        coder.ceval('fclose', fp);
    end
    
    
    if (en && (count < numRecs))
              
        % cache data in memory or use fwrite
        if cacheflag == true
            addr = (count*uint32(vect_size))+1;
            for idx = 1:vect_size
                datastore(addr) = data(idx);
                addr = addr + 1;
            end
            timestore(count+uint32(1))=uint64(timestamp);
        else
            % open file in append mode
            fp = coder.ceval('fopen', [logname,'.bin', int8(0)], ['ab', int8(0)]);
            coder.ceval('fwrite', coder.rref(data), elem_size, vect_size, fp);
            if coder.target('Rtw')
                coder.ceval('fwrite', coder.rref(timestamp), uint32(8), uint32(1), fp);
            end
            coder.ceval('fflush', fp);
            coder.ceval('fclose', fp);
        end
        count = count + uint32(1);
        
    else
        % open file in append mode
        fp = coder.ceval('fopen', [logname,'.bin', int8(0)], ['ab', int8(0)]);            
        coder.ceval('printf',['CLOSING file. count = %d %c' uint8(0)], uint32(count), uint8(10));
        if cacheflag
            for idx=count_prev+1:count
                for idx2=(idx-1)*double(vect_size)+1:(idx-1)*double(vect_size)+double(vect_size)
                    coder.ceval('fwrite', coder.rref(datastore(idx2)), elem_size, uint32(1), fp);
                end
                coder.ceval('fwrite', coder.rref(timestore(idx)), uint32(8), uint32(1), fp);
            end
        end
        coder.ceval('fflush', fp);
        coder.ceval('fclose', fp);
        count_prev=count;
    end
end

% return the size of the element in bytes
    function [elem_size, dtype] = get_elem_size(data)
        switch(class(data))
            case 'double'
                elem_size = 8;
                dtype = 1;
            case 'single'
                elem_size = 4;
                dtype = 2;
            case 'int32'
                elem_size = 4;
                dtype = 3;
            case 'uint32'
                elem_size = 4;
                dtype = 4;
            case 'int16'
                elem_size = 2;
                dtype = 5;
            case 'uint16'
                elem_size = 2;
                dtype = 6;
            case 'int8'
                elem_size = 1;
                dtype = 7;
            case 'uint8'
                elem_size = 1;
                dtype = 8;
            case 'logical'
                elem_size = 1;
                dtype = 9;
            case 'embedded.fi'
                nt = numerictype(data);
                elem_size = 2^ceil(log2(ceil(nt.WordLength / 8)));
                dtype = 10;
        end
        if ~isreal(data)
            elem_size = elem_size*2;
        end
        
        elem_size = uint16(elem_size);
        dtype = uint8(dtype);
    end
end

== matlab function VTOL_v2_r2018b/PX4 SD Card Logger4/SDCard_logger ==
  data: en input boolean; data input; logname parameter uint8; cacheflag parameter boolean; numRecs parameter uint32
%% PX4 SD Card Logger
% Note: All data needs to be of the same type (e.g. double)
% Header information format:
%           String "MWLOG"
%           Time/Date 4 bytes (time())
%           Number of Signals per record Logged 1 byte (256 max)
%           Data Type of Signals Logged  1 byte (1-10)
%           Number of bytes per record 2 bytes (65535 max)
% This does NOT include the number of data sets logged.
% i.e. The Reader is responsible for reading until EOF.
% Steve Kuznicki
% Copyright 2018 The MathWorks, Inc.

function SDCard_logger(en, data, logname, cacheflag, numRecs)

persistent fp count elem_size vect_size datastore timestore count_prev

if coder.target('Rtw')
    
    coder.cinclude('<stdio.h>');
    coder.cinclude('<time.h>');
    
    if coder.target('Rtw')
        coder.cinclude('<drivers/drv_hrt.h>');
    end
    
    if coder.target('Rtw')
        timestamp=coder.opaque('uint64_t');
        timestamp=coder.ceval('hrt_absolute_time');
    else
        timestamp = uint64(0);
    end
    
    if isempty(count)
        count = uint32(0);
        count_prev=count;
        fp = coder.opaque('FILE*', 'NULL');
        if cacheflag == true
            datastore = zeros(numRecs*uint32(coder.const(numel(data))), 1, 'like', data);
            timestore=uint64(zeros(numRecs, 1));
        end
        
        [elsize, eltype] = get_elem_size(data);
        elem_size = coder.const(uint16(elsize));
        elem_type = coder.const(uint8(eltype));
        vect_size = coder.const(uint8(numel(data)));
        coder.ceval('printf',['OPENING file %s vect_size %d elem_size %d numRecs %d %c' uint8(0)], ...
            [logname,'.bin', int8(0)], uint32(vect_size), uint32(elem_size), uint32(numRecs), uint8(10));
        fp = coder.ceval('fopen', [logname,'.bin', int8(0)], ['wb', int8(0)]);
        
        % Write header information here
        % header token + version
        mlStrVer = 'MWLOG';
        coder.ceval('fwrite', coder.rref(mlStrVer), uint32(1), length(mlStrVer), fp);
        % date/time
        tm = uint32(0);
        tmptr = uint32(0);
        tm = coder.ceval('time',coder.wref(tmptr));
        coder.ceval('fwrite', coder.rref(tm), uint32(4), uint32(1), fp);
        % number of elements in each record
        coder.ceval('fwrite', coder.rref(vect_size), uint32(1), uint32(1), fp);
        % data type of the elements
        coder.ceval('fwrite', coder.rref(elem_type), uint32(1), uint32(1), fp);
        % size of each record in bytes
        recSize = elem_size * uint16(vect_size);
        coder.ceval('fwrite', coder.rref(recSize), uint32(2), uint32(1), fp);
        coder.ceval('fclose', fp);
    end
    
    
    if (en && (count < numRecs))
              
        % cache data in memory or use fwrite
        if cacheflag == true
            addr = (count*uint32(vect_size))+1;
            for idx = 1:vect_size
                datastore(addr) = data(idx);
                addr = addr + 1;
            end
            timestore(count+uint32(1))=uint64(timestamp);
        else
            % open file in append mode
            fp = coder.ceval('fopen', [logname,'.bin', int8(0)], ['ab', int8(0)]);
            coder.ceval('fwrite', coder.rref(data), elem_size, vect_size, fp);
            if coder.target('Rtw')
                coder.ceval('fwrite', coder.rref(timestamp), uint32(8), uint32(1), fp);
            end
            coder.ceval('fflush', fp);
            coder.ceval('fclose', fp);
        end
        count = count + uint32(1);
        
    else
        % open file in append mode
        fp = coder.ceval('fopen', [logname,'.bin', int8(0)], ['ab', int8(0)]);            
        coder.ceval('printf',['CLOSING file. count = %d %c' uint8(0)], uint32(count), uint8(10));
        if cacheflag
            for idx=count_prev+1:count
                for idx2=(idx-1)*double(vect_size)+1:(idx-1)*double(vect_size)+double(vect_size)
                    coder.ceval('fwrite', coder.rref(datastore(idx2)), elem_size, uint32(1), fp);
                end
                coder.ceval('fwrite', coder.rref(timestore(idx)), uint32(8), uint32(1), fp);
            end
        end
        coder.ceval('fflush', fp);
        coder.ceval('fclose', fp);
        count_prev=count;
    end
end

% return the size of the element in bytes
    function [elem_size, dtype] = get_elem_size(data)
        switch(class(data))
            case 'double'
                elem_size = 8;
                dtype = 1;
            case 'single'
                elem_size = 4;
                dtype = 2;
            case 'int32'
                elem_size = 4;
                dtype = 3;
            case 'uint32'
                elem_size = 4;
                dtype = 4;
            case 'int16'
                elem_size = 2;
                dtype = 5;
            case 'uint16'
                elem_size = 2;
                dtype = 6;
            case 'int8'
                elem_size = 1;
                dtype = 7;
            case 'uint8'
                elem_size = 1;
                dtype = 8;
            case 'logical'
                elem_size = 1;
                dtype = 9;
            case 'embedded.fi'
                nt = numerictype(data);
                elem_size = 2^ceil(log2(ceil(nt.WordLength / 8)));
                dtype = 10;
        end
        if ~isreal(data)
            elem_size = elem_size*2;
        end
        
        elem_size = uint16(elem_size);
        dtype = uint8(dtype);
    end
end
